simulink model "airspeed_by_pitch_loop"  (R2014b)
settings: Solver=ode45  StartTime=0.0  StopTime=10.0  MaxStep=0.1  RelTol=1e-3
undefined symbols (not defined in the file or in its folder): a_theta_1, a_theta_2, a_theta_3, a_V1, k_d_theta, k_i_V2, k_p_theta, k_p_V2, P
settings Model: Creator=kunalmenda  LastModifiedBy=kunalmenda

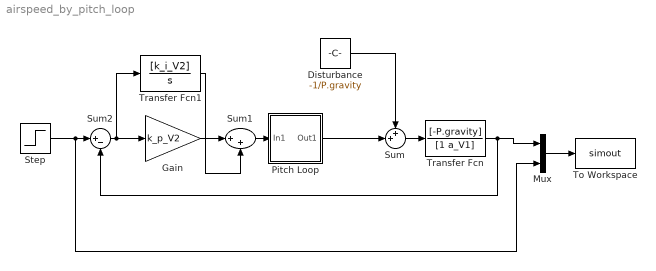
== system airspeed_by_pitch_loop ==
  Disturbance : Constant  Value=-1/P.gravity
  Gain : Gain  Gain=k_p_V2
  Mux : Mux  Inputs=2
  "Pitch Loop " : Subsystem
  Step : Step  After=10  SampleTime=0
  Sum : Sum  Inputs=++|
  Sum1 : Sum  Inputs=|++
  Sum2 : Sum  Inputs=|+-
  To Workspace : ToWorkspace  VariableName=simout  SaveFormat=Timeseries  SampleTime=-1
  Transfer Fcn : TransferFcn  Numerator=[-P.gravity]  Denominator=[1 a_V1]
  Transfer Fcn1 : TransferFcn  Numerator=[k_i_V2]  Denominator=[1 0]
  wires:
  Sum2/1 -> Transfer Fcn1/1, Gain/1
  Step/1 -> Mux/2, Sum2/1
  Mux/1 -> To Workspace/1
  Gain/1 -> Sum1/1
  Transfer Fcn1/1 -> Sum1/2
  Sum1/1 -> "Pitch Loop "/1(In1)
  "Pitch Loop "/1(Out1) -> Sum/2
  Disturbance/1 -> Sum/1
  Sum/1 -> Transfer Fcn/1
  Transfer Fcn/1 -> Sum2/2, Mux/1

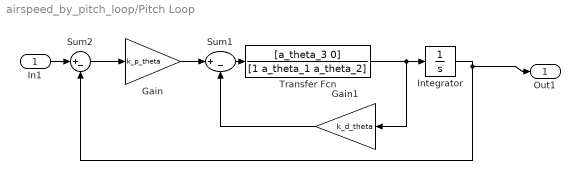
== system airspeed_by_pitch_loop/Pitch Loop  ==
  In1 : Inport
  Gain : Gain  Gain=k_p_theta
  Gain1 : Gain  Gain=k_d_theta
  Integrator : Integrator
  Sum1 : Sum  Inputs=|+-
  Sum2 : Sum  Inputs=|+-
  Transfer Fcn : TransferFcn  Numerator=[a_theta_3 0]  Denominator=[1 a_theta_1 a_theta_2]
  Out1 : Outport
  wires:
  Sum2/1 -> Gain/1
  Transfer Fcn/1 -> Gain1/1, Integrator/1
  Sum1/1 -> Transfer Fcn/1
  Integrator/1 -> Out1/1, Sum2/2
  Gain1/1 -> Sum1/2
  Gain/1 -> Sum1/1
  In1/1 -> Sum2/1
